simulink library "INT_ASDdc_SelectParameter"  (R2016b)
settings: Solver=VariableStepAuto  StartTime=0.0  StopTime=10.0  RelTol=1e-3
settings Model: Creator=lenovo  LastModifiedBy=lenovo

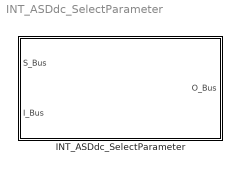
== system INT_ASDdc_SelectParameter ==
  INT_ASDdc_SelectParameter : Subsystem

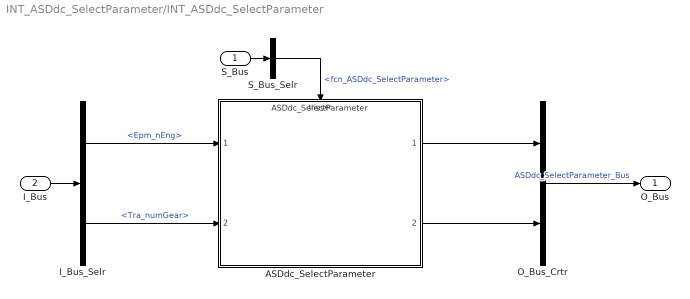
== system INT_ASDdc_SelectParameter/INT_ASDdc_SelectParameter ==
  S_Bus : Inport
  I_Bus : Inport  Port=2
  ASDdc_SelectParameter : ModelReference  ModelNameDialog=ASDdc_SelectParameter  SimulationMode=Normal  ModelReferenceVersion=1.24  TriggerPortName=function  TriggerPortTriggerType=function-call  TriggerPortStatesWhenEnabling=held
  I_Bus_Selr : BusSelector  OutputSignals=Epm_nEng,Tra_numGear
  O_Bus_Crtr : BusCreator  Inputs=2
  S_Bus_Selr : BusSelector  OutputSignals=fcn_ASDdc_SelectParameter
  O_Bus : Outport
  wires:
  S_Bus_Selr/1 -> ASDdc_SelectParameter/Trigger  "<fcn_ASDdc_SelectParameter>"
  S_Bus/1 -> S_Bus_Selr/1
  I_Bus/1 -> I_Bus_Selr/1
  I_Bus_Selr/1 -> ASDdc_SelectParameter/1  "<Epm_nEng>"
  I_Bus_Selr/2 -> ASDdc_SelectParameter/2  "<Tra_numGear>"
  O_Bus_Crtr/1 -> O_Bus/1  "ASDdc_SelectParameter_Bus"
  ASDdc_SelectParameter/1 -> O_Bus_Crtr/1
  ASDdc_SelectParameter/2 -> O_Bus_Crtr/2
